simulink library "Miscellaneous"  (R2023a)
settings: Solver=ode45  StartTime=0.0  StopTime=10.0  RelTol=1e-3  EnableMultiTasking=on
libraries: simulink x4
(part 1 of 2)
settings Model: Creator=N  LastModifiedBy=Jozko Mrkvicka
settings SolverCC: AlgebraicLoopSolver=TrustRegion
settings DataIOCC: LimitDataPoints=on  SaveFormat=Array  ReturnWorkspaceOutputs=off
settings OptimizationCC: LifeSpan=inf
settings DebuggingCC: UnconnectedInputMsg=warning  UnconnectedOutputMsg=warning  UnconnectedLineMsg=warning  SFUnexpectedBacktrackingDiag=warning  SFNoUnconditionalDefaultTransitionDiag=warning  ArithmeticOperatorsInVariantConditions=warning
settings ModelReferenceCC: EnableRefExpFcnMdlSchedulingChecks=on
settings SFSimCC: SimUseLocalCustomCode=off  CustomCodeUndefinedFunction=UseInterfaceOnly
settings RTWCC: RTWUseLocalCustomCode=off
settings CodeAppCC: StateflowObjectComments=on
settings GRTTargetCC: TargetLangStandard=C89/C90 (ANSI)
settings ConfigComp: CovMetricSettings=dw  CovSaveCumulativeToWorkspaceVar=on  CovSaveSingleToWorkspaceVar=on  CovExternalEMLEnable=off

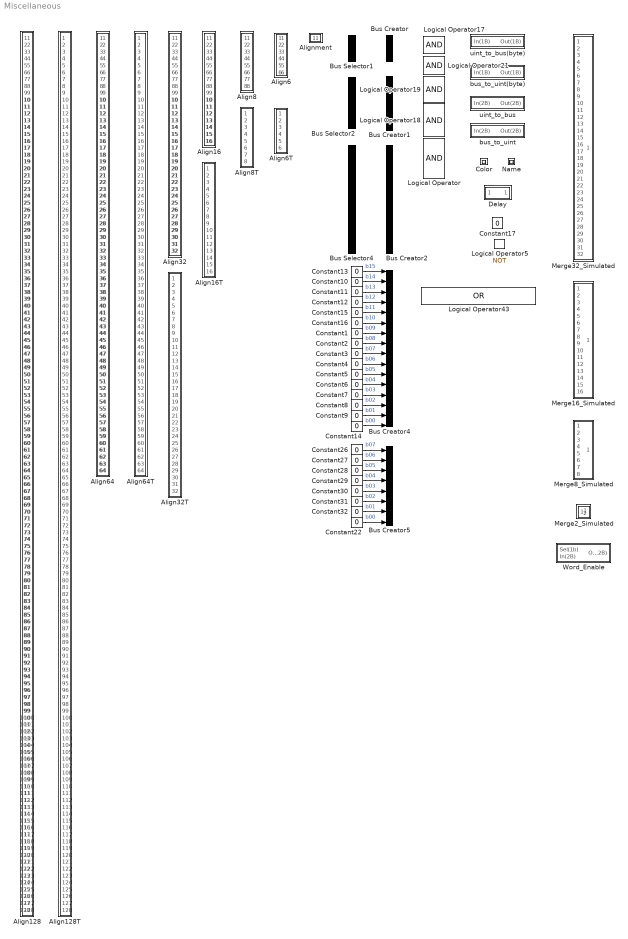
== system Miscellaneous ==
  Align128 : Subsystem
  Align128T : Subsystem
  Align16 : Subsystem
  Align16T : Subsystem
  Align32 : Subsystem
  Align32T : Subsystem
  Align6 : Subsystem
  Align64 : Subsystem
  Align64T : Subsystem
  Align6T : Subsystem
  Align8 : Subsystem
  Align8T : Subsystem
  Alignment : Subsystem
  Bus Creator : BusCreator  Inputs=4
  Bus Creator1 : BusCreator  Inputs=8
  Bus Creator2 : BusCreator  Inputs=16
  Bus Creator4 : BusCreator  Inputs=16
  Bus Creator5 : BusCreator  Inputs=8
  Bus Selector1 : BusSelector  OutputSignals=b3,b2,b1,b0
  Bus Selector2 : BusSelector  OutputSignals=b7,b6,b5,b4,b3,b2,b1,b0
  Bus Selector4 : BusSelector  OutputSignals=b15,b14,b13,b12,b11,b10,b09,b08,b07,b06,b05,b04,b03,b02,b01,b00
  Color : Subsystem
  Constant{1..17,22,26..32} (25 alike) : Constant  Value=0  OutDataTypeStr=boolean
  Delay : Subsystem
  Logical Operator : Logic  Inputs=6  IconShape=distinctive  AllPortsSameDT=off  OutDataTypeStr=boolean
  Logical Operator17 : Logic  IconShape=distinctive  AllPortsSameDT=off  OutDataTypeStr=boolean
  Logical Operator18 : Logic  Inputs=5  IconShape=distinctive  AllPortsSameDT=off  OutDataTypeStr=boolean
  Logical Operator19 : Logic  Inputs=4  IconShape=distinctive  AllPortsSameDT=off  OutDataTypeStr=boolean
  Logical Operator21 : Logic  Inputs=3  IconShape=distinctive  AllPortsSameDT=off  OutDataTypeStr=boolean
  Logical Operator43 : Logic  Operator=OR  Inputs=16  IconShape=distinctive  OutDataTypeStr=boolean
  Logical Operator5 : Logic  Operator=NOT  IconShape=distinctive  AllPortsSameDT=off  OutDataTypeStr=boolean
  Merge16_Simulated : MATLAB Function  TreatAsAtomicUnit=on
      settings: LibrarySourceBlock=Memory_Blocks_Lib/Memory_Blocks_Lib/4096x1B_RAM_Simulated
  Merge2_Simulated : Subsystem
      settings: PortSchema="{\"entries\":[{\"content\":{\"sides\":[{\"content\":{\"connectorIds\":[\"In1\"]},\"type\":\"ConnectorPlacement.EquallySpacedRectSide\",\"uuid\":\"74758995-5ec8-49f8-a534-c3a678c5c312\"},{\"content\":{\"side\":\"RIGHT\"},\"type\":\"ConnectorPlacement.EquallySpacedRectSide\",\"uuid\":\"c467dbeb-9f00-48b9-a78d-a08162163a10\"},{\"content\":{\"connectorIds\":[\"Out1\"],\"side\":\"TOP\"},\"type\":\"ConnectorPlacement.EquallySpacedRectSide\",\"uuid\":\"39dea3b5-6733-4ade-ab22-e62d310be187\"},{\"content\":{\"connectorIds\":[\"In2\"],\"side\":\"BOTTOM\"},\"type\":\"ConnectorPlacement.EquallySpacedRectSide\",\"uuid\":\"73149fc1-24d9-4bdc-92e2-12fb1d742836\"}]},\"type\":\"ConnectorPlacement.EquallySpacedConnector\",\"uuid\":\"fd2226dc-a4d3-43ad-9cda-54babd09ac78\"}],\"packageUris\":[\"http://schema.mathworks.com/mf0/Connector/R2020b\"],\"version\":\"1.0\"}"
  Merge32_Simulated : MATLAB Function  TreatAsAtomicUnit=on
      settings: LibrarySourceBlock=Memory_Blocks_Lib/Memory_Blocks_Lib/4096x1B_RAM_Simulated
  Merge8_Simulated : MATLAB Function  TreatAsAtomicUnit=on
      settings: LibrarySourceBlock=Memory_Blocks_Lib/Memory_Blocks_Lib/4096x1B_RAM_Simulated
  Name : Subsystem
  Word_Enable : Subsystem
  bus_to_uint : Subsystem
  bus_to_uint(byte) : Subsystem
  uint_to_bus : Subsystem
  uint_to_bus(byte) : Subsystem
  wires:
  Constant3/1 -> Bus Creator4/9  "b07"
  Constant16/1 -> Bus Creator4/6  "b10"
  Constant2/1 -> Bus Creator4/8  "b08"
  Constant14/1 -> Bus Creator4/16  "b00"
  Constant7/1 -> Bus Creator4/13  "b03"
  Constant10/1 -> Bus Creator4/2  "b14"
  Constant11/1 -> Bus Creator4/3  "b13"
  Constant12/1 -> Bus Creator4/4  "b12"
  Constant8/1 -> Bus Creator4/14  "b02"
  Constant9/1 -> Bus Creator4/15  "b01"
  Constant5/1 -> Bus Creator4/11  "b05"
  Constant6/1 -> Bus Creator4/12  "b04"
  Constant13/1 -> Bus Creator4/1  "b15"
  Constant4/1 -> Bus Creator4/10  "b06"
  Constant15/1 -> Bus Creator4/5  "b11"
  Constant1/1 -> Bus Creator4/7  "b09"
  Constant32/1 -> Bus Creator5/7  "b01"
  Constant31/1 -> Bus Creator5/6  "b02"
  Constant28/1 -> Bus Creator5/3  "b05"
  Constant27/1 -> Bus Creator5/2  "b06"
  Constant26/1 -> Bus Creator5/1  "b07"
  Constant22/1 -> Bus Creator5/8  "b00"
  Constant30/1 -> Bus Creator5/5  "b03"
  Constant29/1 -> Bus Creator5/4  "b04"

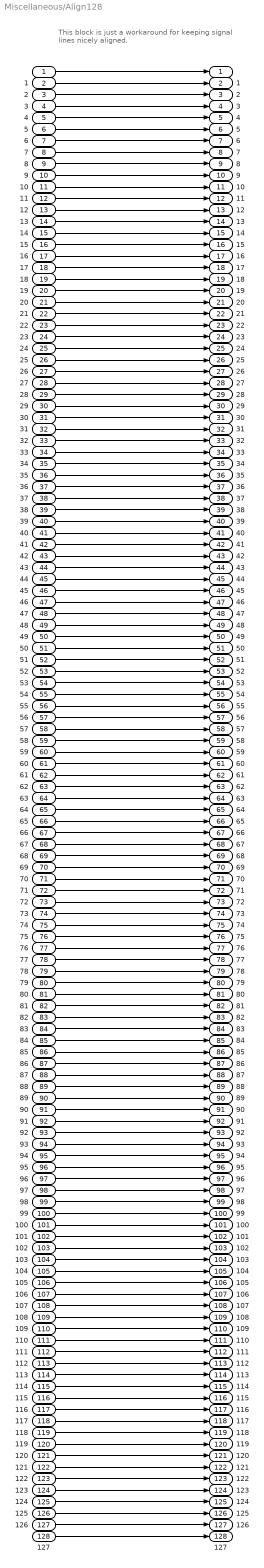
== system Miscellaneous/Align128 ==
  note: This block is just a workaround for keeping signal lines nicely aligned.
  " " : Inport
  " 1" : Inport  Port=2
  " 2" : Inport  Port=3
  " 3" : Inport  Port=4
  " 4" : Inport  Port=5
  " 5" : Inport  Port=6
  " 6" : Inport  Port=7
  " 7" : Inport  Port=8
  " 8" : Inport  Port=9
  " 9" : Inport  Port=10
  " 10" : Inport  Port=11
  " 11" : Inport  Port=12
  " 12" : Inport  Port=13
  " 13" : Inport  Port=14
  " 14" : Inport  Port=15
  " 15" : Inport  Port=16
  " 16" : Inport  Port=17
  " 17" : Inport  Port=18
  " 18" : Inport  Port=19
  " 19" : Inport  Port=20
  " 20" : Inport  Port=21
  " 21" : Inport  Port=22
  " 22" : Inport  Port=23
  " 23" : Inport  Port=24
  " 24" : Inport  Port=25
  " 25" : Inport  Port=26
  " 26" : Inport  Port=27
  " 27" : Inport  Port=28
  " 28" : Inport  Port=29
  " 29" : Inport  Port=30
  " 30" : Inport  Port=31
  " 31" : Inport  Port=32
  " 32" : Inport  Port=33
  " 33" : Inport  Port=34
  " 34" : Inport  Port=35
  " 35" : Inport  Port=36
  " 36" : Inport  Port=37
  " 37" : Inport  Port=38
  " 38" : Inport  Port=39
  " 39" : Inport  Port=40
  " 40" : Inport  Port=41
  " 41" : Inport  Port=42
  " 42" : Inport  Port=43
  " 43" : Inport  Port=44
  " 44" : Inport  Port=45
  " 45" : Inport  Port=46
  " 46" : Inport  Port=47
  " 47" : Inport  Port=48
  " 48" : Inport  Port=49
  " 49" : Inport  Port=50
  " 50" : Inport  Port=51
  " 51" : Inport  Port=52
  " 52" : Inport  Port=53
  " 53" : Inport  Port=54
  " 54" : Inport  Port=55
  " 55" : Inport  Port=56
  " 56" : Inport  Port=57
  " 57" : Inport  Port=58
  " 58" : Inport  Port=59
  " 59" : Inport  Port=60
  " 60" : Inport  Port=61
  " 61" : Inport  Port=62
  " 62" : Inport  Port=63
  " 63" : Inport  Port=64
  " 64" : Inport  Port=65
  " 65" : Inport  Port=66
  " 66" : Inport  Port=67
  " 67" : Inport  Port=68
  " 68" : Inport  Port=69
  " 69" : Inport  Port=70
  " 70" : Inport  Port=71
  " 71" : Inport  Port=72
  " 72" : Inport  Port=73
  " 73" : Inport  Port=74
  " 74" : Inport  Port=75
  " 75" : Inport  Port=76
  " 76" : Inport  Port=77
  " 77" : Inport  Port=78
  " 78" : Inport  Port=79
  " 79" : Inport  Port=80
  " 80" : Inport  Port=81
  " 81" : Inport  Port=82
  " 82" : Inport  Port=83
  " 83" : Inport  Port=84
  " 84" : Inport  Port=85
  " 85" : Inport  Port=86
  " 86" : Inport  Port=87
  " 87" : Inport  Port=88
  " 88" : Inport  Port=89
  " 89" : Inport  Port=90
  " 90" : Inport  Port=91
  " 91" : Inport  Port=92
  " 92" : Inport  Port=93
  " 93" : Inport  Port=94
  " 94" : Inport  Port=95
  " 95" : Inport  Port=96
  " 96" : Inport  Port=97
  " 97" : Inport  Port=98
  " 98" : Inport  Port=99
  " 99" : Inport  Port=100
  " 100" : Inport  Port=101
  " 101" : Inport  Port=102
  " 102" : Inport  Port=103
  " 103" : Inport  Port=104
  " 104" : Inport  Port=105
  " 105" : Inport  Port=106
  " 106" : Inport  Port=107
  " 107" : Inport  Port=108
  " 108" : Inport  Port=109
  " 109" : Inport  Port=110
  " 110" : Inport  Port=111
  " 111" : Inport  Port=112
  " 112" : Inport  Port=113
  " 113" : Inport  Port=114
  " 114" : Inport  Port=115
  " 115" : Inport  Port=116
  " 116" : Inport  Port=117
  " 117" : Inport  Port=118
  " 118" : Inport  Port=119
  " 119" : Inport  Port=120
  " 120" : Inport  Port=121
  " 121" : Inport  Port=122
  " 122" : Inport  Port=123
  " 123" : Inport  Port=124
  " 124" : Inport  Port=125
  " 125" : Inport  Port=126
  " 126" : Inport  Port=127
  " 127" : Inport  Port=128
  "  " : Outport
  "  1" : Outport  Port=2
  "  2" : Outport  Port=3
  "  3" : Outport  Port=4
  "  4" : Outport  Port=5
  "  5" : Outport  Port=6
  "  6" : Outport  Port=7
  "  7" : Outport  Port=8
  "  8" : Outport  Port=9
  "  9" : Outport  Port=10
  "  10" : Outport  Port=11
  "  11" : Outport  Port=12
  "  12" : Outport  Port=13
  "  13" : Outport  Port=14
  "  14" : Outport  Port=15
  "  15" : Outport  Port=16
  "  16" : Outport  Port=17
  "  17" : Outport  Port=18
  "  18" : Outport  Port=19
  "  19" : Outport  Port=20
  "  20" : Outport  Port=21
  "  21" : Outport  Port=22
  "  22" : Outport  Port=23
  "  23" : Outport  Port=24
  "  24" : Outport  Port=25
  "  25" : Outport  Port=26
  "  26" : Outport  Port=27
  "  27" : Outport  Port=28
  "  28" : Outport  Port=29
  "  29" : Outport  Port=30
  "  30" : Outport  Port=31
  "  31" : Outport  Port=32
  "  32" : Outport  Port=33
  "  33" : Outport  Port=34
  "  34" : Outport  Port=35
  "  35" : Outport  Port=36
  "  36" : Outport  Port=37
  "  37" : Outport  Port=38
  "  38" : Outport  Port=39
  "  39" : Outport  Port=40
  "  40" : Outport  Port=41
  "  41" : Outport  Port=42
  "  42" : Outport  Port=43
  "  43" : Outport  Port=44
  "  44" : Outport  Port=45
  "  45" : Outport  Port=46
  "  46" : Outport  Port=47
  "  47" : Outport  Port=48
  "  48" : Outport  Port=49
  "  49" : Outport  Port=50
  "  50" : Outport  Port=51
  "  51" : Outport  Port=52
  "  52" : Outport  Port=53
  "  53" : Outport  Port=54
  "  54" : Outport  Port=55
  "  55" : Outport  Port=56
  "  56" : Outport  Port=57
  "  57" : Outport  Port=58
  "  58" : Outport  Port=59
  "  59" : Outport  Port=60
  "  60" : Outport  Port=61
  "  61" : Outport  Port=62
  "  62" : Outport  Port=63
  "  63" : Outport  Port=64
  "  64" : Outport  Port=65
  "  65" : Outport  Port=66
  "  66" : Outport  Port=67
  "  67" : Outport  Port=68
  "  68" : Outport  Port=69
  "  69" : Outport  Port=70
  "  70" : Outport  Port=71
  "  71" : Outport  Port=72
  "  72" : Outport  Port=73
  "  73" : Outport  Port=74
  "  74" : Outport  Port=75
  "  75" : Outport  Port=76
  "  76" : Outport  Port=77
  "  77" : Outport  Port=78
  "  78" : Outport  Port=79
  "  79" : Outport  Port=80
  "  80" : Outport  Port=81
  "  81" : Outport  Port=82
  "  82" : Outport  Port=83
  "  83" : Outport  Port=84
  "  84" : Outport  Port=85
  "  85" : Outport  Port=86
  "  86" : Outport  Port=87
  "  87" : Outport  Port=88
  "  88" : Outport  Port=89
  "  89" : Outport  Port=90
  "  90" : Outport  Port=91
  "  91" : Outport  Port=92
  "  92" : Outport  Port=93
  "  93" : Outport  Port=94
  "  94" : Outport  Port=95
  "  95" : Outport  Port=96
  "  96" : Outport  Port=97
  "  97" : Outport  Port=98
  "  98" : Outport  Port=99
  "  99" : Outport  Port=100
  "  100" : Outport  Port=101
  "  101" : Outport  Port=102
  "  102" : Outport  Port=103
  "  103" : Outport  Port=104
  "  104" : Outport  Port=105
  "  105" : Outport  Port=106
  "  106" : Outport  Port=107
  "  107" : Outport  Port=108
  "  108" : Outport  Port=109
  "  109" : Outport  Port=110
  "  110" : Outport  Port=111
  "  111" : Outport  Port=112
  "  112" : Outport  Port=113
  "  113" : Outport  Port=114
  "  114" : Outport  Port=115
  "  115" : Outport  Port=116
  "  116" : Outport  Port=117
  "  117" : Outport  Port=118
  "  118" : Outport  Port=119
  "  119" : Outport  Port=120
  "  120" : Outport  Port=121
  "  121" : Outport  Port=122
  "  122" : Outport  Port=123
  "  123" : Outport  Port=124
  "  124" : Outport  Port=125
  "  125" : Outport  Port=126
  "  126" : Outport  Port=127
  "  127" : Outport  Port=128
  wires:
  " "/1 -> "  "/1
  " 1"/1 -> "  1"/1
  " 2"/1 -> "  2"/1
  " 3"/1 -> "  3"/1
  " 4"/1 -> "  4"/1
  " 5"/1 -> "  5"/1
  " 6"/1 -> "  6"/1
  " 7"/1 -> "  7"/1
  " 8"/1 -> "  8"/1
  " 9"/1 -> "  9"/1
  " 10"/1 -> "  10"/1
  " 11"/1 -> "  11"/1
  " 12"/1 -> "  12"/1
  " 13"/1 -> "  13"/1
  " 14"/1 -> "  14"/1
  " 15"/1 -> "  15"/1
  " 16"/1 -> "  16"/1
  " 17"/1 -> "  17"/1
  " 18"/1 -> "  18"/1
  " 19"/1 -> "  19"/1
  " 20"/1 -> "  20"/1
  " 21"/1 -> "  21"/1
  " 22"/1 -> "  22"/1
  " 23"/1 -> "  23"/1
  " 24"/1 -> "  24"/1
  " 25"/1 -> "  25"/1
  " 26"/1 -> "  26"/1
  " 27"/1 -> "  27"/1
  " 28"/1 -> "  28"/1
  " 29"/1 -> "  29"/1
  " 30"/1 -> "  30"/1
  " 31"/1 -> "  31"/1
  " 32"/1 -> "  32"/1
  " 33"/1 -> "  33"/1
  " 34"/1 -> "  34"/1
  " 35"/1 -> "  35"/1
  " 36"/1 -> "  36"/1
  " 37"/1 -> "  37"/1
  " 38"/1 -> "  38"/1
  " 39"/1 -> "  39"/1
  " 40"/1 -> "  40"/1
  " 41"/1 -> "  41"/1
  " 42"/1 -> "  42"/1
  " 43"/1 -> "  43"/1
  " 44"/1 -> "  44"/1
  " 45"/1 -> "  45"/1
  " 46"/1 -> "  46"/1
  " 47"/1 -> "  47"/1
  " 48"/1 -> "  48"/1
  " 49"/1 -> "  49"/1
  " 50"/1 -> "  50"/1
  " 51"/1 -> "  51"/1
  " 52"/1 -> "  52"/1
  " 53"/1 -> "  53"/1
  " 54"/1 -> "  54"/1
  " 55"/1 -> "  55"/1
  " 56"/1 -> "  56"/1
  " 57"/1 -> "  57"/1
  " 58"/1 -> "  58"/1
  " 59"/1 -> "  59"/1
  " 60"/1 -> "  60"/1
  " 61"/1 -> "  61"/1
  " 62"/1 -> "  62"/1
  " 63"/1 -> "  63"/1
  " 64"/1 -> "  64"/1
  " 65"/1 -> "  65"/1
  " 66"/1 -> "  66"/1
  " 67"/1 -> "  67"/1
  " 68"/1 -> "  68"/1
  " 69"/1 -> "  69"/1
  " 70"/1 -> "  70"/1
  " 71"/1 -> "  71"/1
  " 72"/1 -> "  72"/1
  " 73"/1 -> "  73"/1
  " 74"/1 -> "  74"/1
  " 75"/1 -> "  75"/1
  " 76"/1 -> "  76"/1
  " 77"/1 -> "  77"/1
  " 78"/1 -> "  78"/1
  " 79"/1 -> "  79"/1
  " 80"/1 -> "  80"/1
  " 81"/1 -> "  81"/1
  " 82"/1 -> "  82"/1
  " 83"/1 -> "  83"/1
  " 84"/1 -> "  84"/1
  " 85"/1 -> "  85"/1
  " 86"/1 -> "  86"/1
  " 87"/1 -> "  87"/1
  " 88"/1 -> "  88"/1
  " 89"/1 -> "  89"/1
  " 90"/1 -> "  90"/1
  " 91"/1 -> "  91"/1
  " 92"/1 -> "  92"/1
  " 93"/1 -> "  93"/1
  " 94"/1 -> "  94"/1
  " 95"/1 -> "  95"/1
  " 96"/1 -> "  96"/1
  " 97"/1 -> "  97"/1
  " 98"/1 -> "  98"/1
  " 99"/1 -> "  99"/1
  " 100"/1 -> "  100"/1
  " 101"/1 -> "  101"/1
  " 102"/1 -> "  102"/1
  " 103"/1 -> "  103"/1
  " 104"/1 -> "  104"/1
  " 105"/1 -> "  105"/1
  " 106"/1 -> "  106"/1
  " 107"/1 -> "  107"/1
  " 108"/1 -> "  108"/1
  " 109"/1 -> "  109"/1
  " 110"/1 -> "  110"/1
  " 111"/1 -> "  111"/1
  " 112"/1 -> "  112"/1
  " 113"/1 -> "  113"/1
  " 114"/1 -> "  114"/1
  " 115"/1 -> "  115"/1
  " 116"/1 -> "  116"/1
  " 117"/1 -> "  117"/1
  " 118"/1 -> "  118"/1
  " 119"/1 -> "  119"/1
  " 120"/1 -> "  120"/1
  " 121"/1 -> "  121"/1
  " 122"/1 -> "  122"/1
  " 123"/1 -> "  123"/1
  " 124"/1 -> "  124"/1
  " 125"/1 -> "  125"/1
  " 126"/1 -> "  126"/1
  " 127"/1 -> "  127"/1

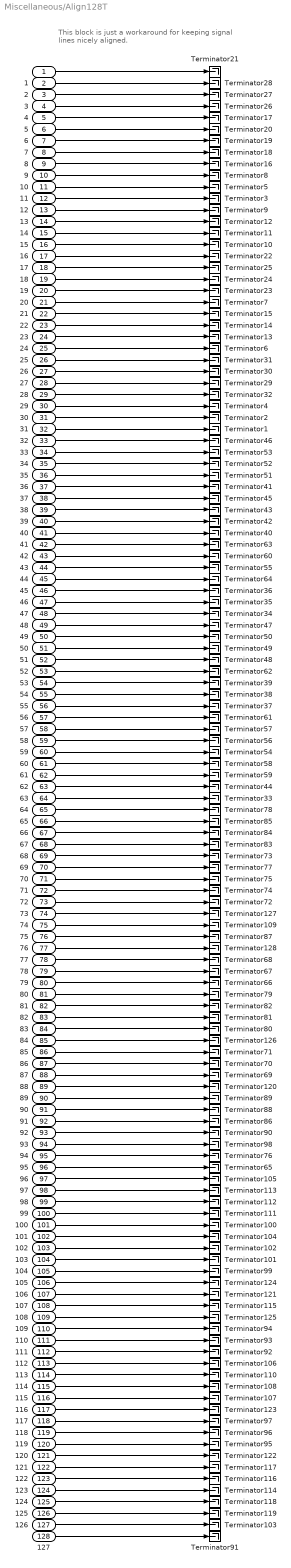
== system Miscellaneous/Align128T ==
  note: This block is just a workaround for keeping signal lines nicely aligned.
  " " : Inport
  " 1" : Inport  Port=2
  " 2" : Inport  Port=3
  " 3" : Inport  Port=4
  " 4" : Inport  Port=5
  " 5" : Inport  Port=6
  " 6" : Inport  Port=7
  " 7" : Inport  Port=8
  " 8" : Inport  Port=9
  " 9" : Inport  Port=10
  " 10" : Inport  Port=11
  " 11" : Inport  Port=12
  " 12" : Inport  Port=13
  " 13" : Inport  Port=14
  " 14" : Inport  Port=15
  " 15" : Inport  Port=16
  " 16" : Inport  Port=17
  " 17" : Inport  Port=18
  " 18" : Inport  Port=19
  " 19" : Inport  Port=20
  " 20" : Inport  Port=21
  " 21" : Inport  Port=22
  " 22" : Inport  Port=23
  " 23" : Inport  Port=24
  " 24" : Inport  Port=25
  " 25" : Inport  Port=26
  " 26" : Inport  Port=27
  " 27" : Inport  Port=28
  " 28" : Inport  Port=29
  " 29" : Inport  Port=30
  " 30" : Inport  Port=31
  " 31" : Inport  Port=32
  " 32" : Inport  Port=33
  " 33" : Inport  Port=34
  " 34" : Inport  Port=35
  " 35" : Inport  Port=36
  " 36" : Inport  Port=37
  " 37" : Inport  Port=38
  " 38" : Inport  Port=39
  " 39" : Inport  Port=40
  " 40" : Inport  Port=41
  " 41" : Inport  Port=42
  " 42" : Inport  Port=43
  " 43" : Inport  Port=44
  " 44" : Inport  Port=45
  " 45" : Inport  Port=46
  " 46" : Inport  Port=47
  " 47" : Inport  Port=48
  " 48" : Inport  Port=49
  " 49" : Inport  Port=50
  " 50" : Inport  Port=51
  " 51" : Inport  Port=52
  " 52" : Inport  Port=53
  " 53" : Inport  Port=54
  " 54" : Inport  Port=55
  " 55" : Inport  Port=56
  " 56" : Inport  Port=57
  " 57" : Inport  Port=58
  " 58" : Inport  Port=59
  " 59" : Inport  Port=60
  " 60" : Inport  Port=61
  " 61" : Inport  Port=62
  " 62" : Inport  Port=63
  " 63" : Inport  Port=64
  " 64" : Inport  Port=65
  " 65" : Inport  Port=66
  " 66" : Inport  Port=67
  " 67" : Inport  Port=68
  " 68" : Inport  Port=69
  " 69" : Inport  Port=70
  " 70" : Inport  Port=71
  " 71" : Inport  Port=72
  " 72" : Inport  Port=73
  " 73" : Inport  Port=74
  " 74" : Inport  Port=75
  " 75" : Inport  Port=76
  " 76" : Inport  Port=77
  " 77" : Inport  Port=78
  " 78" : Inport  Port=79
  " 79" : Inport  Port=80
  " 80" : Inport  Port=81
  " 81" : Inport  Port=82
  " 82" : Inport  Port=83
  " 83" : Inport  Port=84
  " 84" : Inport  Port=85
  " 85" : Inport  Port=86
  " 86" : Inport  Port=87
  " 87" : Inport  Port=88
  " 88" : Inport  Port=89
  " 89" : Inport  Port=90
  " 90" : Inport  Port=91
  " 91" : Inport  Port=92
  " 92" : Inport  Port=93
  " 93" : Inport  Port=94
  " 94" : Inport  Port=95
  " 95" : Inport  Port=96
  " 96" : Inport  Port=97
  " 97" : Inport  Port=98
  " 98" : Inport  Port=99
  " 99" : Inport  Port=100
  " 100" : Inport  Port=101
  " 101" : Inport  Port=102
  " 102" : Inport  Port=103
  " 103" : Inport  Port=104
  " 104" : Inport  Port=105
  " 105" : Inport  Port=106
  " 106" : Inport  Port=107
  " 107" : Inport  Port=108
  " 108" : Inport  Port=109
  " 109" : Inport  Port=110
  " 110" : Inport  Port=111
  " 111" : Inport  Port=112
  " 112" : Inport  Port=113
  " 113" : Inport  Port=114
  " 114" : Inport  Port=115
  " 115" : Inport  Port=116
  " 116" : Inport  Port=117
  " 117" : Inport  Port=118
  " 118" : Inport  Port=119
  " 119" : Inport  Port=120
  " 120" : Inport  Port=121
  " 121" : Inport  Port=122
  " 122" : Inport  Port=123
  " 123" : Inport  Port=124
  " 124" : Inport  Port=125
  " 125" : Inport  Port=126
  " 126" : Inport  Port=127
  " 127" : Inport  Port=128
  Terminator{1..128} (128 alike) : Terminator
  wires:
  " "/1 -> Terminator21/1
  " 1"/1 -> Terminator28/1
  " 2"/1 -> Terminator27/1
  " 3"/1 -> Terminator26/1
  " 4"/1 -> Terminator17/1
  " 5"/1 -> Terminator20/1
  " 6"/1 -> Terminator19/1
  " 7"/1 -> Terminator18/1
  " 8"/1 -> Terminator16/1
  " 9"/1 -> Terminator8/1
  " 10"/1 -> Terminator5/1
  " 11"/1 -> Terminator3/1
  " 12"/1 -> Terminator9/1
  " 13"/1 -> Terminator12/1
  " 14"/1 -> Terminator11/1
  " 15"/1 -> Terminator10/1
  " 16"/1 -> Terminator22/1
  " 17"/1 -> Terminator25/1
  " 18"/1 -> Terminator24/1
  " 19"/1 -> Terminator23/1
  " 20"/1 -> Terminator7/1
  " 21"/1 -> Terminator15/1
  " 22"/1 -> Terminator14/1
  " 23"/1 -> Terminator13/1
  " 24"/1 -> Terminator6/1
  " 25"/1 -> Terminator31/1
  " 26"/1 -> Terminator30/1
  " 27"/1 -> Terminator29/1
  " 28"/1 -> Terminator32/1
  " 29"/1 -> Terminator4/1
  " 30"/1 -> Terminator2/1
  " 31"/1 -> Terminator1/1
  " 32"/1 -> Terminator46/1
  " 33"/1 -> Terminator53/1
  " 34"/1 -> Terminator52/1
  " 35"/1 -> Terminator51/1
  " 36"/1 -> Terminator41/1
  " 37"/1 -> Terminator45/1
  " 38"/1 -> Terminator43/1
  " 39"/1 -> Terminator42/1
  " 40"/1 -> Terminator40/1
  " 41"/1 -> Terminator63/1
  " 42"/1 -> Terminator60/1
  " 43"/1 -> Terminator55/1
  " 44"/1 -> Terminator64/1
  " 45"/1 -> Terminator36/1
  " 46"/1 -> Terminator35/1
  " 47"/1 -> Terminator34/1
  " 48"/1 -> Terminator47/1
  " 49"/1 -> Terminator50/1
  " 50"/1 -> Terminator49/1
  " 51"/1 -> Terminator48/1
  " 52"/1 -> Terminator62/1
  " 53"/1 -> Terminator39/1
  " 54"/1 -> Terminator38/1
  " 55"/1 -> Terminator37/1
  " 56"/1 -> Terminator61/1
  " 57"/1 -> Terminator57/1
  " 58"/1 -> Terminator56/1
  " 59"/1 -> Terminator54/1
  " 60"/1 -> Terminator58/1
  " 61"/1 -> Terminator59/1
  " 62"/1 -> Terminator44/1
  " 63"/1 -> Terminator33/1
  " 64"/1 -> Terminator78/1
  " 65"/1 -> Terminator85/1
  " 66"/1 -> Terminator84/1
  " 67"/1 -> Terminator83/1
  " 68"/1 -> Terminator73/1
  " 69"/1 -> Terminator77/1
  " 70"/1 -> Terminator75/1
  " 71"/1 -> Terminator74/1
  " 72"/1 -> Terminator72/1
  " 73"/1 -> Terminator127/1
  " 74"/1 -> Terminator109/1
  " 75"/1 -> Terminator87/1
  " 76"/1 -> Terminator128/1
  " 77"/1 -> Terminator68/1
  " 78"/1 -> Terminator67/1
  " 79"/1 -> Terminator66/1
  " 80"/1 -> Terminator79/1
  " 81"/1 -> Terminator82/1
  " 82"/1 -> Terminator81/1
  " 83"/1 -> Terminator80/1
  " 84"/1 -> Terminator126/1
  " 85"/1 -> Terminator71/1
  " 86"/1 -> Terminator70/1
  " 87"/1 -> Terminator69/1
  " 88"/1 -> Terminator120/1
  " 89"/1 -> Terminator89/1
  " 90"/1 -> Terminator88/1
  " 91"/1 -> Terminator86/1
  " 92"/1 -> Terminator90/1
  " 93"/1 -> Terminator98/1
  " 94"/1 -> Terminator76/1
  " 95"/1 -> Terminator65/1
  " 96"/1 -> Terminator105/1
  " 97"/1 -> Terminator113/1
  " 98"/1 -> Terminator112/1
  " 99"/1 -> Terminator111/1
  " 100"/1 -> Terminator100/1
  " 101"/1 -> Terminator104/1
  " 102"/1 -> Terminator102/1
  " 103"/1 -> Terminator101/1
  " 104"/1 -> Terminator99/1
  " 105"/1 -> Terminator124/1
  " 106"/1 -> Terminator121/1
  " 107"/1 -> Terminator115/1
  " 108"/1 -> Terminator125/1
  " 109"/1 -> Terminator94/1
  " 110"/1 -> Terminator93/1
  " 111"/1 -> Terminator92/1
  " 112"/1 -> Terminator106/1
  " 113"/1 -> Terminator110/1
  " 114"/1 -> Terminator108/1
  " 115"/1 -> Terminator107/1
  " 116"/1 -> Terminator123/1
  " 117"/1 -> Terminator97/1
  " 118"/1 -> Terminator96/1
  " 119"/1 -> Terminator95/1
  " 120"/1 -> Terminator122/1
  " 121"/1 -> Terminator117/1
  " 122"/1 -> Terminator116/1
  " 123"/1 -> Terminator114/1
  " 124"/1 -> Terminator118/1
  " 125"/1 -> Terminator119/1
  " 126"/1 -> Terminator103/1
  " 127"/1 -> Terminator91/1

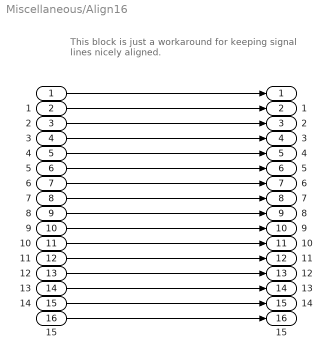
== system Miscellaneous/Align16 ==
  note: This block is just a workaround for keeping signal lines nicely aligned.
  " " : Inport
  " 1" : Inport  Port=2
  " 2" : Inport  Port=3
  " 3" : Inport  Port=4
  " 4" : Inport  Port=5
  " 5" : Inport  Port=6
  " 6" : Inport  Port=7
  " 7" : Inport  Port=8
  " 8" : Inport  Port=9
  " 9" : Inport  Port=10
  " 10" : Inport  Port=11
  " 11" : Inport  Port=12
  " 12" : Inport  Port=13
  " 13" : Inport  Port=14
  " 14" : Inport  Port=15
  " 15" : Inport  Port=16
  "  " : Outport
  "  1" : Outport  Port=2
  "  2" : Outport  Port=3
  "  3" : Outport  Port=4
  "  4" : Outport  Port=5
  "  5" : Outport  Port=6
  "  6" : Outport  Port=7
  "  7" : Outport  Port=8
  "  8" : Outport  Port=9
  "  9" : Outport  Port=10
  "  10" : Outport  Port=11
  "  11" : Outport  Port=12
  "  12" : Outport  Port=13
  "  13" : Outport  Port=14
  "  14" : Outport  Port=15
  "  15" : Outport  Port=16
  wires:
  " "/1 -> "  "/1
  " 1"/1 -> "  1"/1
  " 2"/1 -> "  2"/1
  " 3"/1 -> "  3"/1
  " 4"/1 -> "  4"/1
  " 5"/1 -> "  5"/1
  " 6"/1 -> "  6"/1
  " 7"/1 -> "  7"/1
  " 8"/1 -> "  8"/1
  " 9"/1 -> "  9"/1
  " 10"/1 -> "  10"/1
  " 11"/1 -> "  11"/1
  " 12"/1 -> "  12"/1
  " 13"/1 -> "  13"/1
  " 14"/1 -> "  14"/1
  " 15"/1 -> "  15"/1

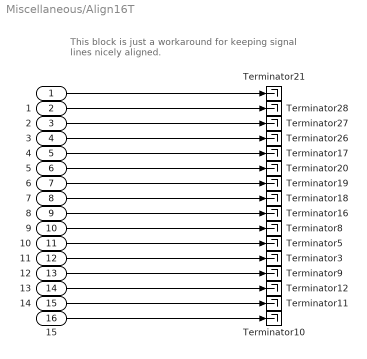
== system Miscellaneous/Align16T ==
  note: This block is just a workaround for keeping signal lines nicely aligned.
  " " : Inport
  " 1" : Inport  Port=2
  " 2" : Inport  Port=3
  " 3" : Inport  Port=4
  " 4" : Inport  Port=5
  " 5" : Inport  Port=6
  " 6" : Inport  Port=7
  " 7" : Inport  Port=8
  " 8" : Inport  Port=9
  " 9" : Inport  Port=10
  " 10" : Inport  Port=11
  " 11" : Inport  Port=12
  " 12" : Inport  Port=13
  " 13" : Inport  Port=14
  " 14" : Inport  Port=15
  " 15" : Inport  Port=16
  Terminator{3,5,8..12,16..21,26..28} (16 alike) : Terminator
  wires:
  " "/1 -> Terminator21/1
  " 1"/1 -> Terminator28/1
  " 2"/1 -> Terminator27/1
  " 3"/1 -> Terminator26/1
  " 4"/1 -> Terminator17/1
  " 5"/1 -> Terminator20/1
  " 6"/1 -> Terminator19/1
  " 7"/1 -> Terminator18/1
  " 8"/1 -> Terminator16/1
  " 9"/1 -> Terminator8/1
  " 10"/1 -> Terminator5/1
  " 11"/1 -> Terminator3/1
  " 12"/1 -> Terminator9/1
  " 13"/1 -> Terminator12/1
  " 14"/1 -> Terminator11/1
  " 15"/1 -> Terminator10/1

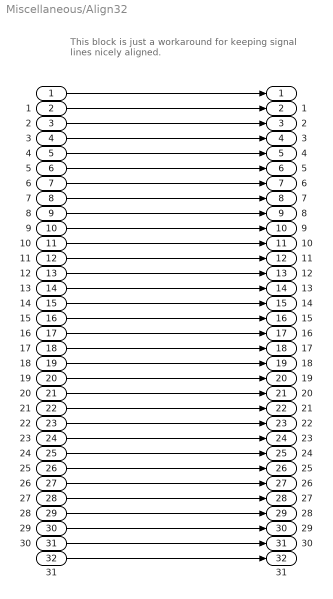
== system Miscellaneous/Align32 ==
  note: This block is just a workaround for keeping signal lines nicely aligned.
  " " : Inport
  " 1" : Inport  Port=2
  " 2" : Inport  Port=3
  " 3" : Inport  Port=4
  " 4" : Inport  Port=5
  " 5" : Inport  Port=6
  " 6" : Inport  Port=7
  " 7" : Inport  Port=8
  " 8" : Inport  Port=9
  " 9" : Inport  Port=10
  " 10" : Inport  Port=11
  " 11" : Inport  Port=12
  " 12" : Inport  Port=13
  " 13" : Inport  Port=14
  " 14" : Inport  Port=15
  " 15" : Inport  Port=16
  " 16" : Inport  Port=17
  " 17" : Inport  Port=18
  " 18" : Inport  Port=19
  " 19" : Inport  Port=20
  " 20" : Inport  Port=21
  " 21" : Inport  Port=22
  " 22" : Inport  Port=23
  " 23" : Inport  Port=24
  " 24" : Inport  Port=25
  " 25" : Inport  Port=26
  " 26" : Inport  Port=27
  " 27" : Inport  Port=28
  " 28" : Inport  Port=29
  " 29" : Inport  Port=30
  " 30" : Inport  Port=31
  " 31" : Inport  Port=32
  "  " : Outport
  "  1" : Outport  Port=2
  "  2" : Outport  Port=3
  "  3" : Outport  Port=4
  "  4" : Outport  Port=5
  "  5" : Outport  Port=6
  "  6" : Outport  Port=7
  "  7" : Outport  Port=8
  "  8" : Outport  Port=9
  "  9" : Outport  Port=10
  "  10" : Outport  Port=11
  "  11" : Outport  Port=12
  "  12" : Outport  Port=13
  "  13" : Outport  Port=14
  "  14" : Outport  Port=15
  "  15" : Outport  Port=16
  "  16" : Outport  Port=17
  "  17" : Outport  Port=18
  "  18" : Outport  Port=19
  "  19" : Outport  Port=20
  "  20" : Outport  Port=21
  "  21" : Outport  Port=22
  "  22" : Outport  Port=23
  "  23" : Outport  Port=24
  "  24" : Outport  Port=25
  "  25" : Outport  Port=26
  "  26" : Outport  Port=27
  "  27" : Outport  Port=28
  "  28" : Outport  Port=29
  "  29" : Outport  Port=30
  "  30" : Outport  Port=31
  "  31" : Outport  Port=32
  wires:
  " "/1 -> "  "/1
  " 1"/1 -> "  1"/1
  " 2"/1 -> "  2"/1
  " 3"/1 -> "  3"/1
  " 4"/1 -> "  4"/1
  " 5"/1 -> "  5"/1
  " 6"/1 -> "  6"/1
  " 7"/1 -> "  7"/1
  " 8"/1 -> "  8"/1
  " 9"/1 -> "  9"/1
  " 10"/1 -> "  10"/1
  " 11"/1 -> "  11"/1
  " 12"/1 -> "  12"/1
  " 13"/1 -> "  13"/1
  " 14"/1 -> "  14"/1
  " 15"/1 -> "  15"/1
  " 16"/1 -> "  16"/1
  " 17"/1 -> "  17"/1
  " 18"/1 -> "  18"/1
  " 19"/1 -> "  19"/1
  " 20"/1 -> "  20"/1
  " 21"/1 -> "  21"/1
  " 22"/1 -> "  22"/1
  " 23"/1 -> "  23"/1
  " 24"/1 -> "  24"/1
  " 25"/1 -> "  25"/1
  " 26"/1 -> "  26"/1
  " 27"/1 -> "  27"/1
  " 28"/1 -> "  28"/1
  " 29"/1 -> "  29"/1
  " 30"/1 -> "  30"/1
  " 31"/1 -> "  31"/1

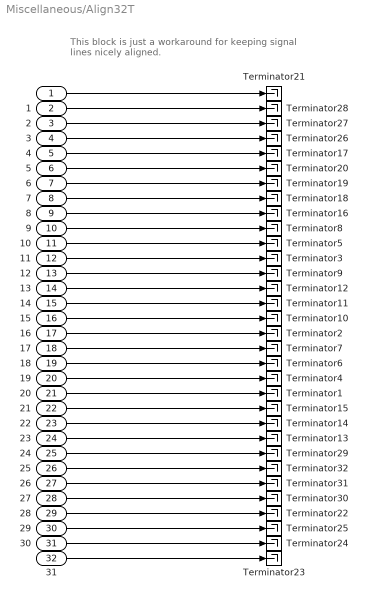
== system Miscellaneous/Align32T ==
  note: This block is just a workaround for keeping signal lines nicely aligned.
  " " : Inport
  " 1" : Inport  Port=2
  " 2" : Inport  Port=3
  " 3" : Inport  Port=4
  " 4" : Inport  Port=5
  " 5" : Inport  Port=6
  " 6" : Inport  Port=7
  " 7" : Inport  Port=8
  " 8" : Inport  Port=9
  " 9" : Inport  Port=10
  " 10" : Inport  Port=11
  " 11" : Inport  Port=12
  " 12" : Inport  Port=13
  " 13" : Inport  Port=14
  " 14" : Inport  Port=15
  " 15" : Inport  Port=16
  " 16" : Inport  Port=17
  " 17" : Inport  Port=18
  " 18" : Inport  Port=19
  " 19" : Inport  Port=20
  " 20" : Inport  Port=21
  " 21" : Inport  Port=22
  " 22" : Inport  Port=23
  " 23" : Inport  Port=24
  " 24" : Inport  Port=25
  " 25" : Inport  Port=26
  " 26" : Inport  Port=27
  " 27" : Inport  Port=28
  " 28" : Inport  Port=29
  " 29" : Inport  Port=30
  " 30" : Inport  Port=31
  " 31" : Inport  Port=32
  Terminator{1..32} (32 alike) : Terminator
  wires:
  " "/1 -> Terminator21/1
  " 1"/1 -> Terminator28/1
  " 2"/1 -> Terminator27/1
  " 3"/1 -> Terminator26/1
  " 4"/1 -> Terminator17/1
  " 5"/1 -> Terminator20/1
  " 6"/1 -> Terminator19/1
  " 7"/1 -> Terminator18/1
  " 8"/1 -> Terminator16/1
  " 9"/1 -> Terminator8/1
  " 10"/1 -> Terminator5/1
  " 11"/1 -> Terminator3/1
  " 12"/1 -> Terminator9/1
  " 13"/1 -> Terminator12/1
  " 14"/1 -> Terminator11/1
  " 15"/1 -> Terminator10/1
  " 16"/1 -> Terminator2/1
  " 17"/1 -> Terminator7/1
  " 18"/1 -> Terminator6/1
  " 19"/1 -> Terminator4/1
  " 20"/1 -> Terminator1/1
  " 21"/1 -> Terminator15/1
  " 22"/1 -> Terminator14/1
  " 23"/1 -> Terminator13/1
  " 24"/1 -> Terminator29/1
  " 25"/1 -> Terminator32/1
  " 26"/1 -> Terminator31/1
  " 27"/1 -> Terminator30/1
  " 28"/1 -> Terminator22/1
  " 29"/1 -> Terminator25/1
  " 30"/1 -> Terminator24/1
  " 31"/1 -> Terminator23/1

== system Miscellaneous/Align6 ==
  note: This block is just a workaround for keeping signal lines nicely aligned.
  " " : Inport
  " 1" : Inport  Port=2
  " 2" : Inport  Port=3
  " 3" : Inport  Port=4
  " 4" : Inport  Port=5
  " 5" : Inport  Port=6
  "  " : Outport
  "  1" : Outport  Port=2
  "  2" : Outport  Port=3
  "  3" : Outport  Port=4
  "  4" : Outport  Port=5
  "  5" : Outport  Port=6
  wires:
  " "/1 -> "  "/1
  " 1"/1 -> "  1"/1
  " 2"/1 -> "  2"/1
  " 3"/1 -> "  3"/1
  " 4"/1 -> "  4"/1
  " 5"/1 -> "  5"/1

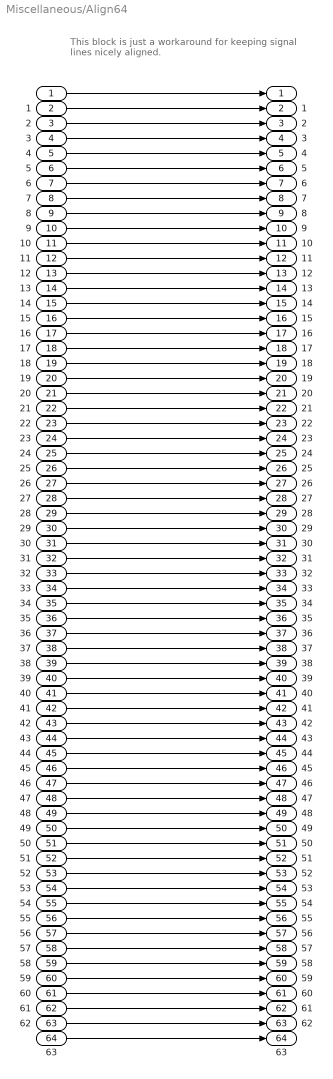
== system Miscellaneous/Align64 ==
  note: This block is just a workaround for keeping signal lines nicely aligned.
  " " : Inport
  " 1" : Inport  Port=2
  " 2" : Inport  Port=3
  " 3" : Inport  Port=4
  " 4" : Inport  Port=5
  " 5" : Inport  Port=6
  " 6" : Inport  Port=7
  " 7" : Inport  Port=8
  " 8" : Inport  Port=9
  " 9" : Inport  Port=10
  " 10" : Inport  Port=11
  " 11" : Inport  Port=12
  " 12" : Inport  Port=13
  " 13" : Inport  Port=14
  " 14" : Inport  Port=15
  " 15" : Inport  Port=16
  " 16" : Inport  Port=17
  " 17" : Inport  Port=18
  " 18" : Inport  Port=19
  " 19" : Inport  Port=20
  " 20" : Inport  Port=21
  " 21" : Inport  Port=22
  " 22" : Inport  Port=23
  " 23" : Inport  Port=24
  " 24" : Inport  Port=25
  " 25" : Inport  Port=26
  " 26" : Inport  Port=27
  " 27" : Inport  Port=28
  " 28" : Inport  Port=29
  " 29" : Inport  Port=30
  " 30" : Inport  Port=31
  " 31" : Inport  Port=32
  " 32" : Inport  Port=33
  " 33" : Inport  Port=34
  " 34" : Inport  Port=35
  " 35" : Inport  Port=36
  " 36" : Inport  Port=37
  " 37" : Inport  Port=38
  " 38" : Inport  Port=39
  " 39" : Inport  Port=40
  " 40" : Inport  Port=41
  " 41" : Inport  Port=42
  " 42" : Inport  Port=43
  " 43" : Inport  Port=44
  " 44" : Inport  Port=45
  " 45" : Inport  Port=46
  " 46" : Inport  Port=47
  " 47" : Inport  Port=48
  " 48" : Inport  Port=49
  " 49" : Inport  Port=50
  " 50" : Inport  Port=51
  " 51" : Inport  Port=52
  " 52" : Inport  Port=53
  " 53" : Inport  Port=54
  " 54" : Inport  Port=55
  " 55" : Inport  Port=56
  " 56" : Inport  Port=57
  " 57" : Inport  Port=58
  " 58" : Inport  Port=59
  " 59" : Inport  Port=60
  " 60" : Inport  Port=61
  " 61" : Inport  Port=62
  " 62" : Inport  Port=63
  " 63" : Inport  Port=64
  "  " : Outport
  "  1" : Outport  Port=2
  "  2" : Outport  Port=3
  "  3" : Outport  Port=4
  "  4" : Outport  Port=5
  "  5" : Outport  Port=6
  "  6" : Outport  Port=7
  "  7" : Outport  Port=8
  "  8" : Outport  Port=9
  "  9" : Outport  Port=10
  "  10" : Outport  Port=11
  "  11" : Outport  Port=12
  "  12" : Outport  Port=13
  "  13" : Outport  Port=14
  "  14" : Outport  Port=15
  "  15" : Outport  Port=16
  "  16" : Outport  Port=17
  "  17" : Outport  Port=18
  "  18" : Outport  Port=19
  "  19" : Outport  Port=20
  "  20" : Outport  Port=21
  "  21" : Outport  Port=22
  "  22" : Outport  Port=23
  "  23" : Outport  Port=24
  "  24" : Outport  Port=25
  "  25" : Outport  Port=26
  "  26" : Outport  Port=27
  "  27" : Outport  Port=28
  "  28" : Outport  Port=29
  "  29" : Outport  Port=30
  "  30" : Outport  Port=31
  "  31" : Outport  Port=32
  "  32" : Outport  Port=33
  "  33" : Outport  Port=34
  "  34" : Outport  Port=35
  "  35" : Outport  Port=36
  "  36" : Outport  Port=37
  "  37" : Outport  Port=38
  "  38" : Outport  Port=39
  "  39" : Outport  Port=40
  "  40" : Outport  Port=41
  "  41" : Outport  Port=42
  "  42" : Outport  Port=43
  "  43" : Outport  Port=44
  "  44" : Outport  Port=45
  "  45" : Outport  Port=46
  "  46" : Outport  Port=47
  "  47" : Outport  Port=48
  "  48" : Outport  Port=49
  "  49" : Outport  Port=50
  "  50" : Outport  Port=51
  "  51" : Outport  Port=52
  "  52" : Outport  Port=53
  "  53" : Outport  Port=54
  "  54" : Outport  Port=55
  "  55" : Outport  Port=56
  "  56" : Outport  Port=57
  "  57" : Outport  Port=58
  "  58" : Outport  Port=59
  "  59" : Outport  Port=60
  "  60" : Outport  Port=61
  "  61" : Outport  Port=62
  "  62" : Outport  Port=63
  "  63" : Outport  Port=64
  wires:
  " "/1 -> "  "/1
  " 1"/1 -> "  1"/1
  " 2"/1 -> "  2"/1
  " 3"/1 -> "  3"/1
  " 4"/1 -> "  4"/1
  " 5"/1 -> "  5"/1
  " 6"/1 -> "  6"/1
  " 7"/1 -> "  7"/1
  " 8"/1 -> "  8"/1
  " 9"/1 -> "  9"/1
  " 10"/1 -> "  10"/1
  " 11"/1 -> "  11"/1
  " 12"/1 -> "  12"/1
  " 13"/1 -> "  13"/1
  " 14"/1 -> "  14"/1
  " 15"/1 -> "  15"/1
  " 16"/1 -> "  16"/1
  " 17"/1 -> "  17"/1
  " 18"/1 -> "  18"/1
  " 19"/1 -> "  19"/1
  " 20"/1 -> "  20"/1
  " 21"/1 -> "  21"/1
  " 22"/1 -> "  22"/1
  " 23"/1 -> "  23"/1
  " 24"/1 -> "  24"/1
  " 25"/1 -> "  25"/1
  " 26"/1 -> "  26"/1
  " 27"/1 -> "  27"/1
  " 28"/1 -> "  28"/1
  " 29"/1 -> "  29"/1
  " 30"/1 -> "  30"/1
  " 31"/1 -> "  31"/1
  " 32"/1 -> "  32"/1
  " 33"/1 -> "  33"/1
  " 34"/1 -> "  34"/1
  " 35"/1 -> "  35"/1
  " 36"/1 -> "  36"/1
  " 37"/1 -> "  37"/1
  " 38"/1 -> "  38"/1
  " 39"/1 -> "  39"/1
  " 40"/1 -> "  40"/1
  " 41"/1 -> "  41"/1
  " 42"/1 -> "  42"/1
  " 43"/1 -> "  43"/1
  " 44"/1 -> "  44"/1
  " 45"/1 -> "  45"/1
  " 46"/1 -> "  46"/1
  " 47"/1 -> "  47"/1
  " 48"/1 -> "  48"/1
  " 49"/1 -> "  49"/1
  " 50"/1 -> "  50"/1
  " 51"/1 -> "  51"/1
  " 52"/1 -> "  52"/1
  " 53"/1 -> "  53"/1
  " 54"/1 -> "  54"/1
  " 55"/1 -> "  55"/1
  " 56"/1 -> "  56"/1
  " 57"/1 -> "  57"/1
  " 58"/1 -> "  58"/1
  " 59"/1 -> "  59"/1
  " 60"/1 -> "  60"/1
  " 61"/1 -> "  61"/1
  " 62"/1 -> "  62"/1
  " 63"/1 -> "  63"/1

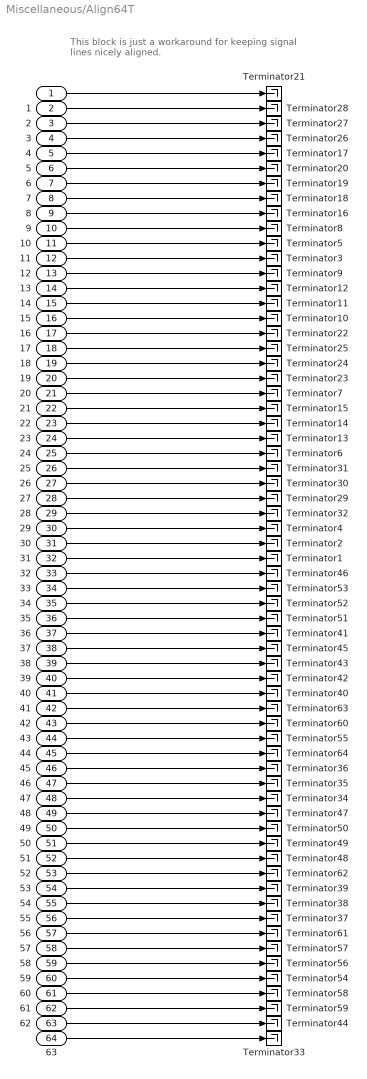
== system Miscellaneous/Align64T ==
  note: This block is just a workaround for keeping signal lines nicely aligned.
  " " : Inport
  " 1" : Inport  Port=2
  " 2" : Inport  Port=3
  " 3" : Inport  Port=4
  " 4" : Inport  Port=5
  " 5" : Inport  Port=6
  " 6" : Inport  Port=7
  " 7" : Inport  Port=8
  " 8" : Inport  Port=9
  " 9" : Inport  Port=10
  " 10" : Inport  Port=11
  " 11" : Inport  Port=12
  " 12" : Inport  Port=13
  " 13" : Inport  Port=14
  " 14" : Inport  Port=15
  " 15" : Inport  Port=16
  " 16" : Inport  Port=17
  " 17" : Inport  Port=18
  " 18" : Inport  Port=19
  " 19" : Inport  Port=20
  " 20" : Inport  Port=21
  " 21" : Inport  Port=22
  " 22" : Inport  Port=23
  " 23" : Inport  Port=24
  " 24" : Inport  Port=25
  " 25" : Inport  Port=26
  " 26" : Inport  Port=27
  " 27" : Inport  Port=28
  " 28" : Inport  Port=29
  " 29" : Inport  Port=30
  " 30" : Inport  Port=31
  " 31" : Inport  Port=32
  " 32" : Inport  Port=33
  " 33" : Inport  Port=34
  " 34" : Inport  Port=35
  " 35" : Inport  Port=36
  " 36" : Inport  Port=37
  " 37" : Inport  Port=38
  " 38" : Inport  Port=39
  " 39" : Inport  Port=40
  " 40" : Inport  Port=41
  " 41" : Inport  Port=42
  " 42" : Inport  Port=43
  " 43" : Inport  Port=44
  " 44" : Inport  Port=45
  " 45" : Inport  Port=46
  " 46" : Inport  Port=47
  " 47" : Inport  Port=48
  " 48" : Inport  Port=49
  " 49" : Inport  Port=50
  " 50" : Inport  Port=51
  " 51" : Inport  Port=52
  " 52" : Inport  Port=53
  " 53" : Inport  Port=54
  " 54" : Inport  Port=55
  " 55" : Inport  Port=56
  " 56" : Inport  Port=57
  " 57" : Inport  Port=58
  " 58" : Inport  Port=59
  " 59" : Inport  Port=60
  " 60" : Inport  Port=61
  " 61" : Inport  Port=62
  " 62" : Inport  Port=63
  " 63" : Inport  Port=64
  Terminator{1..64} (64 alike) : Terminator
  wires:
  " "/1 -> Terminator21/1
  " 1"/1 -> Terminator28/1
  " 2"/1 -> Terminator27/1
  " 3"/1 -> Terminator26/1
  " 4"/1 -> Terminator17/1
  " 5"/1 -> Terminator20/1
  " 6"/1 -> Terminator19/1
  " 7"/1 -> Terminator18/1
  " 8"/1 -> Terminator16/1
  " 9"/1 -> Terminator8/1
  " 10"/1 -> Terminator5/1
  " 11"/1 -> Terminator3/1
  " 12"/1 -> Terminator9/1
  " 13"/1 -> Terminator12/1
  " 14"/1 -> Terminator11/1
  " 15"/1 -> Terminator10/1
  " 16"/1 -> Terminator22/1
  " 17"/1 -> Terminator25/1
  " 18"/1 -> Terminator24/1
  " 19"/1 -> Terminator23/1
  " 20"/1 -> Terminator7/1
  " 21"/1 -> Terminator15/1
  " 22"/1 -> Terminator14/1
  " 23"/1 -> Terminator13/1
  " 24"/1 -> Terminator6/1
  " 25"/1 -> Terminator31/1
  " 26"/1 -> Terminator30/1
  " 27"/1 -> Terminator29/1
  " 28"/1 -> Terminator32/1
  " 29"/1 -> Terminator4/1
  " 30"/1 -> Terminator2/1
  " 31"/1 -> Terminator1/1
  " 32"/1 -> Terminator46/1
  " 33"/1 -> Terminator53/1
  " 34"/1 -> Terminator52/1
  " 35"/1 -> Terminator51/1
  " 36"/1 -> Terminator41/1
  " 37"/1 -> Terminator45/1
  " 38"/1 -> Terminator43/1
  " 39"/1 -> Terminator42/1
  " 40"/1 -> Terminator40/1
  " 41"/1 -> Terminator63/1
  " 42"/1 -> Terminator60/1
  " 43"/1 -> Terminator55/1
  " 44"/1 -> Terminator64/1
  " 45"/1 -> Terminator36/1
  " 46"/1 -> Terminator35/1
  " 47"/1 -> Terminator34/1
  " 48"/1 -> Terminator47/1
  " 49"/1 -> Terminator50/1
  " 50"/1 -> Terminator49/1
  " 51"/1 -> Terminator48/1
  " 52"/1 -> Terminator62/1
  " 53"/1 -> Terminator39/1
  " 54"/1 -> Terminator38/1
  " 55"/1 -> Terminator37/1
  " 56"/1 -> Terminator61/1
  " 57"/1 -> Terminator57/1
  " 58"/1 -> Terminator56/1
  " 59"/1 -> Terminator54/1
  " 60"/1 -> Terminator58/1
  " 61"/1 -> Terminator59/1
  " 62"/1 -> Terminator44/1
  " 63"/1 -> Terminator33/1

== system Miscellaneous/Align6T ==
  note: This block is just a workaround for keeping signal lines nicely aligned.
  " " : Inport
  " 1" : Inport  Port=2
  " 2" : Inport  Port=3
  " 3" : Inport  Port=4
  " 4" : Inport  Port=5
  " 5" : Inport  Port=6
  Terminator{17,20..21,26..28} (6 alike) : Terminator
  wires:
  " "/1 -> Terminator21/1
  " 1"/1 -> Terminator28/1
  " 2"/1 -> Terminator27/1
  " 3"/1 -> Terminator26/1
  " 4"/1 -> Terminator17/1
  " 5"/1 -> Terminator20/1

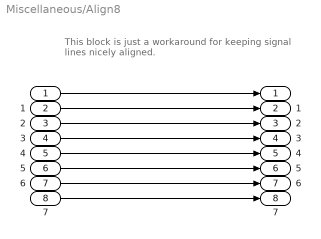
== system Miscellaneous/Align8 ==
  note: This block is just a workaround for keeping signal lines nicely aligned.
  " " : Inport
  " 1" : Inport  Port=2
  " 2" : Inport  Port=3
  " 3" : Inport  Port=4
  " 4" : Inport  Port=5
  " 5" : Inport  Port=6
  " 6" : Inport  Port=7
  " 7" : Inport  Port=8
  "  " : Outport
  "  1" : Outport  Port=2
  "  2" : Outport  Port=3
  "  3" : Outport  Port=4
  "  4" : Outport  Port=5
  "  5" : Outport  Port=6
  "  6" : Outport  Port=7
  "  7" : Outport  Port=8
  wires:
  " "/1 -> "  "/1
  " 1"/1 -> "  1"/1
  " 2"/1 -> "  2"/1
  " 3"/1 -> "  3"/1
  " 4"/1 -> "  4"/1
  " 5"/1 -> "  5"/1
  " 6"/1 -> "  6"/1
  " 7"/1 -> "  7"/1

== system Miscellaneous/Align8T ==
  note: This block is just a workaround for keeping signal lines nicely aligned.
  " " : Inport
  " 1" : Inport  Port=2
  " 2" : Inport  Port=3
  " 3" : Inport  Port=4
  " 4" : Inport  Port=5
  " 5" : Inport  Port=6
  " 6" : Inport  Port=7
  " 7" : Inport  Port=8
  Terminator{17..21,26..28} (8 alike) : Terminator
  wires:
  " "/1 -> Terminator21/1
  " 1"/1 -> Terminator28/1
  " 2"/1 -> Terminator27/1
  " 3"/1 -> Terminator26/1
  " 4"/1 -> Terminator17/1
  " 5"/1 -> Terminator20/1
  " 6"/1 -> Terminator19/1
  " 7"/1 -> Terminator18/1

== system Miscellaneous/Alignment ==
  note: This block is just a workaround for keeping signal lines nicely aligned.
  " " : Inport
  "  " : Outport
  wires:
  " "/1 -> "  "/1

== system Miscellaneous/Color ==
  note: This block is just a workaround for changing color of a line which is connected to it (Simulink does not allow to assign colors to particular lines).
  " " : Inport
  "  " : Outport
  wires:
  " "/1 -> "  "/1

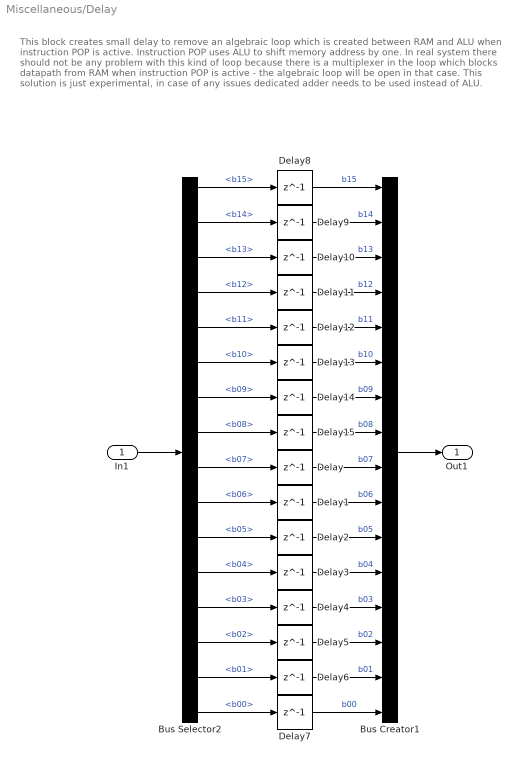
== system Miscellaneous/Delay ==
  note: This block creates small delay to remove an algebraic loop which is created between RAM and ALU when instruction POP is active. Instruction POP uses ALU to shift memory address by one. In real system there should not be any problem with this kind of loop because there is a multiplexer in the loop which blocks datapath from RAM when instruction POP is active - the algebraic loop will be open in that case.
      | This solution is just experimental, in case of any issues dedicated adder needs to be used instead of ALU.
  In1 : Inport
  Bus Creator1 : BusCreator  Inputs=16
  Bus Selector2 : BusSelector  OutputSignals=b15,b14,b13,b12,b11,b10,b09,b08,b07,b06,b05,b04,b03,b02,b01,b00
  Delay{,1..15} (16 alike) : Delay  DelayLength=1  InitialCondition=0
  Out1 : Outport
  wires:
  Delay/1 -> Bus Creator1/9  "b07"
  Delay1/1 -> Bus Creator1/10  "b06"
  Delay2/1 -> Bus Creator1/11  "b05"
  Delay3/1 -> Bus Creator1/12  "b04"
  Delay4/1 -> Bus Creator1/13  "b03"
  Delay5/1 -> Bus Creator1/14  "b02"
  Delay6/1 -> Bus Creator1/15  "b01"
  Delay7/1 -> Bus Creator1/16  "b00"
  Bus Creator1/1 -> Out1/1
  In1/1 -> Bus Selector2/1
  Delay8/1 -> Bus Creator1/1  "b15"
  Delay9/1 -> Bus Creator1/2  "b14"
  Delay10/1 -> Bus Creator1/3  "b13"
  Delay11/1 -> Bus Creator1/4  "b12"
  Delay12/1 -> Bus Creator1/5  "b11"
  Delay13/1 -> Bus Creator1/6  "b10"
  Delay14/1 -> Bus Creator1/7  "b09"
  Delay15/1 -> Bus Creator1/8  "b08"
  Bus Selector2/1 -> Delay8/1  "<b15>"
  Bus Selector2/2 -> Delay9/1  "<b14>"
  Bus Selector2/3 -> Delay10/1  "<b13>"
  Bus Selector2/4 -> Delay11/1  "<b12>"
  Bus Selector2/5 -> Delay12/1  "<b11>"
  Bus Selector2/6 -> Delay13/1  "<b10>"
  Bus Selector2/7 -> Delay14/1  "<b09>"
  Bus Selector2/8 -> Delay15/1  "<b08>"
  Bus Selector2/9 -> Delay/1  "<b07>"
  Bus Selector2/10 -> Delay1/1  "<b06>"
  Bus Selector2/11 -> Delay2/1  "<b05>"
  Bus Selector2/12 -> Delay3/1  "<b04>"
  Bus Selector2/13 -> Delay4/1  "<b03>"
  Bus Selector2/14 -> Delay5/1  "<b02>"
  Bus Selector2/15 -> Delay6/1  "<b01>"
  Bus Selector2/16 -> Delay7/1  "<b00>"

== system Miscellaneous/Merge2_Simulated ==
  Data_1 : Inport  OutDataTypeStr=Bus: BUS_UINT16_T
  Data_0 : Inport  Port=2  OutDataTypeStr=Bus: BUS_UINT16_T
  Merge_Simulated1 : MATLAB Function  TreatAsAtomicUnit=on
      settings: LibrarySourceBlock=Memory_Blocks_Lib/Memory_Blocks_Lib/4096x1B_RAM_Simulated
  DataOut : Outport  OutDataTypeStr=Bus: BUS_UINT16_T
  wires:
  Data_0/1 -> Merge_Simulated1/2(Data_0)
  Data_1/1 -> Merge_Simulated1/1(Data_1)
  Merge_Simulated1/1(DataOut) -> DataOut/1

== system Miscellaneous/Name ==
  note: This block is just a workaround for changing name of a signal which is connected to it (Simulink does not allow to assign multiple signals with the same name to the one bus creator block).
  " " : Inport
  Logical Operator : Logic  Inputs=1  IconShape=distinctive  AllPortsSameDT=off  OutDataTypeStr=boolean
  "  " : Outport
  wires:
  " "/1 -> Logical Operator/1
  Logical Operator/1 -> "  "/1

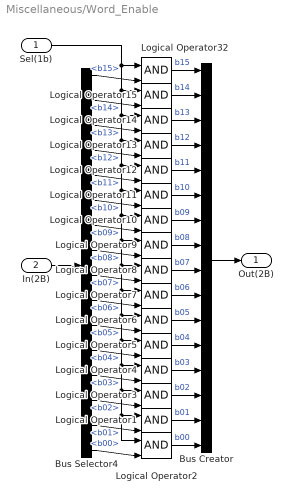
== system Miscellaneous/Word_Enable ==
  Sel(1b) : Inport
  In(2B) : Inport  Port=2
  Bus Creator : BusCreator  Inputs=16
  Bus Selector4 : BusSelector  OutputSignals=b15,b14,b13,b12,b11,b10,b09,b08,b07,b06,b05,b04,b03,b02,b01,b00
  Logical Operator{1..15,32} (16 alike) : Logic  IconShape=distinctive  AllPortsSameDT=off  OutDataTypeStr=boolean
  Out(2B) : Outport  OutputWhenDisabled=reset
  wires:
  Bus Creator/1 -> Out(2B)/1
  In(2B)/1 -> Bus Selector4/1
  Sel(1b)/1 -> Logical Operator32/1, Logical Operator2/1, Logical Operator1/1, Logical Operator3/1, Logical Operator4/1, Logical Operator5/1, Logical Operator6/1, Logical Operator7/1, Logical Operator8/1, Logical Operator9/1, Logical Operator10/1, Logical Operator11/1, Logical Operator12/1, Logical Operator13/1, Logical Operator14/1, Logical Operator15/1
  Bus Selector4/1 -> Logical Operator32/2  "<b15>"
  Bus Selector4/2 -> Logical Operator15/2  "<b14>"
  Bus Selector4/3 -> Logical Operator14/2  "<b13>"
  Bus Selector4/4 -> Logical Operator13/2  "<b12>"
  Bus Selector4/5 -> Logical Operator12/2  "<b11>"
  Bus Selector4/6 -> Logical Operator11/2  "<b10>"
  Bus Selector4/7 -> Logical Operator10/2  "<b09>"
  Bus Selector4/8 -> Logical Operator9/2  "<b08>"
  Bus Selector4/9 -> Logical Operator8/2  "<b07>"
  Bus Selector4/10 -> Logical Operator7/2  "<b06>"
  Bus Selector4/11 -> Logical Operator6/2  "<b05>"
  Bus Selector4/12 -> Logical Operator5/2  "<b04>"
  Bus Selector4/13 -> Logical Operator4/2  "<b03>"
  Bus Selector4/14 -> Logical Operator3/2  "<b02>"
  Bus Selector4/15 -> Logical Operator1/2  "<b01>"
  Bus Selector4/16 -> Logical Operator2/2  "<b00>"
  Logical Operator4/1 -> Bus Creator/13  "b03"
  Logical Operator12/1 -> Bus Creator/5  "b11"
  Logical Operator7/1 -> Bus Creator/10  "b06"
  Logical Operator2/1 -> Bus Creator/16  "b00"
  Logical Operator32/1 -> Bus Creator/1  "b15"
  Logical Operator6/1 -> Bus Creator/11  "b05"
  Logical Operator1/1 -> Bus Creator/15  "b01"
  Logical Operator10/1 -> Bus Creator/7  "b09"
  Logical Operator15/1 -> Bus Creator/2  "b14"
  Logical Operator14/1 -> Bus Creator/3  "b13"
  Logical Operator5/1 -> Bus Creator/12  "b04"
  Logical Operator11/1 -> Bus Creator/6  "b10"
  Logical Operator3/1 -> Bus Creator/14  "b02"
  Logical Operator9/1 -> Bus Creator/8  "b08"
  Logical Operator13/1 -> Bus Creator/4  "b12"
  Logical Operator8/1 -> Bus Creator/9  "b07"

== system Miscellaneous/bus_to_uint ==
  In(2B) : Inport
  Bit to Integer Converter3 : simulink/Logic and Bit Operations/Bit to Integer Converter  nbits=16  bitOrder=MSB first  signedOutputValues=Unsigned  outDtype=uint16  outDtypeSigned=Inherit via internal rule
      settings: LibrarySourceBlock=|
      | commutil2/Bit to Integer
      | Converter
  Bus Selector3 : BusSelector  OutputSignals=b15,b14,b13,b12,b11,b10,b09,b08,b07,b06,b05,b04,b03,b02,b01,b00
  Mux : Mux  Inputs=16
  Out(2B) : Outport
  wires:
  In(2B)/1 -> Bus Selector3/1
  Bit to Integer Converter3/1 -> Out(2B)/1
  Bus Selector3/1 -> Mux/1  "<b15>"
  Bus Selector3/2 -> Mux/2  "<b14>"
  Bus Selector3/3 -> Mux/3  "<b13>"
  Bus Selector3/4 -> Mux/4  "<b12>"
  Bus Selector3/5 -> Mux/5  "<b11>"
  Bus Selector3/6 -> Mux/6  "<b10>"
  Bus Selector3/7 -> Mux/7  "<b09>"
  Bus Selector3/8 -> Mux/8  "<b08>"
  Bus Selector3/10 -> Mux/10  "<b06>"
  Bus Selector3/9 -> Mux/9  "<b07>"
  Bus Selector3/11 -> Mux/11  "<b05>"
  Bus Selector3/12 -> Mux/12  "<b04>"
  Bus Selector3/13 -> Mux/13  "<b03>"
  Bus Selector3/14 -> Mux/14  "<b02>"
  Bus Selector3/15 -> Mux/15  "<b01>"
  Bus Selector3/16 -> Mux/16  "<b00>"
  Mux/1 -> Bit to Integer Converter3/1

== system Miscellaneous/bus_to_uint(byte) ==
  In(1B) : Inport
  Bit to Integer Converter3 : simulink/Logic and Bit Operations/Bit to Integer Converter  nbits=8  bitOrder=MSB first  signedOutputValues=Unsigned  outDtype=uint8  outDtypeSigned=Inherit via internal rule
      settings: LibrarySourceBlock=|
      | commutil2/Bit to Integer
      | Converter
  Bus Selector : BusSelector  OutputSignals=signal1,signal2,signal3,signal4,signal5,signal6,signal7,signal8
  Mux : Mux  Inputs=8
  Out(1B) : Outport
  wires:
  In(1B)/1 -> Bus Selector/1
  Bit to Integer Converter3/1 -> Out(1B)/1
  Mux/1 -> Bit to Integer Converter3/1
  Bus Selector/1 -> Mux/1  "<signal1>"
  Bus Selector/2 -> Mux/2  "<signal2>"
  Bus Selector/3 -> Mux/3  "<signal3>"
  Bus Selector/4 -> Mux/4  "<signal4>"
  Bus Selector/5 -> Mux/5  "<signal5>"
  Bus Selector/6 -> Mux/6  "<signal6>"
  Bus Selector/7 -> Mux/7  "<signal7>"
  Bus Selector/8 -> Mux/8  "<signal8>"

== system Miscellaneous/uint_to_bus ==
  In(2B) : Inport
  Bus Creator : BusCreator  Inputs=16
  Demux2 : Demux  Outputs=16
  Integer to Bit Converter2 : simulink/Logic and Bit Operations/Integer to Bit Converter  nbits=16  signedInputValues=Unsigned  bitOrder=MSB first  outDtype=boolean
      settings: LibrarySourceBlock=|
      | commutil2/Integer to Bit
      | Converter
  Out(2B) : Outport  OutDataTypeStr=boolean
  wires:
  In(2B)/1 -> Integer to Bit Converter2/1
  Bus Creator/1 -> Out(2B)/1
  Demux2/13 -> Bus Creator/13  "b03"
  Demux2/1 -> Bus Creator/1  "b15"
  Demux2/5 -> Bus Creator/5  "b11"
  Demux2/16 -> Bus Creator/16  "b00"
  Demux2/3 -> Bus Creator/3  "b13"
  Demux2/11 -> Bus Creator/11  "b05"
  Demux2/12 -> Bus Creator/12  "b04"
  Demux2/15 -> Bus Creator/15  "b01"
  Demux2/14 -> Bus Creator/14  "b02"
  Demux2/2 -> Bus Creator/2  "b14"
  Demux2/6 -> Bus Creator/6  "b10"
  Demux2/9 -> Bus Creator/9  "b07"
  Demux2/10 -> Bus Creator/10  "b06"
  Demux2/4 -> Bus Creator/4  "b12"
  Demux2/7 -> Bus Creator/7  "b09"
  Demux2/8 -> Bus Creator/8  "b08"
  Integer to Bit Converter2/1 -> Demux2/1

== system Miscellaneous/uint_to_bus(byte) ==
  In(1B) : Inport
  Bus Creator : BusCreator  Inputs=8
  Demux2 : Demux  Outputs=8
  Integer to Bit Converter2 : simulink/Logic and Bit Operations/Integer to Bit Converter  nbits=8  signedInputValues=Unsigned  bitOrder=MSB first  outDtype=boolean
      settings: LibrarySourceBlock=|
      | commutil2/Integer to Bit
      | Converter
  Out(1B) : Outport
  wires:
  In(1B)/1 -> Integer to Bit Converter2/1
  Bus Creator/1 -> Out(1B)/1
  Integer to Bit Converter2/1 -> Demux2/1
  Demux2/1 -> Bus Creator/1  "b7"
  Demux2/2 -> Bus Creator/2  "b6"
  Demux2/3 -> Bus Creator/3  "b5"
  Demux2/4 -> Bus Creator/4  "b4"
  Demux2/5 -> Bus Creator/5  "b3"
  Demux2/6 -> Bus Creator/6  "b2"
  Demux2/7 -> Bus Creator/7  "b1"
  Demux2/8 -> Bus Creator/8  "b0"
